simulink model "s5"  (R2023b)
settings: Solver=ode45  StartTime=3  StopTime=10  RelTol=1e-3
settings Model: Creator=t3  LastModifiedBy=t3

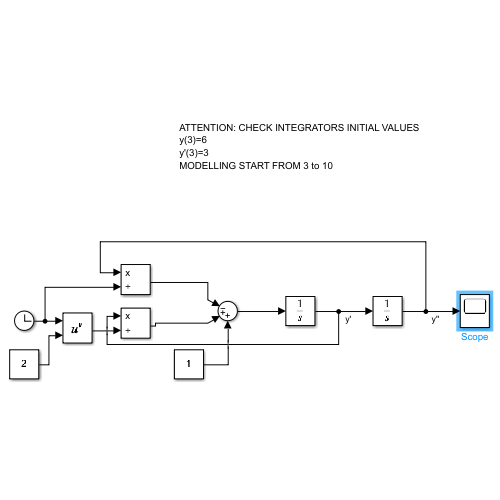
[thumbnail: Simulink's stored preview of the top-level diagram]
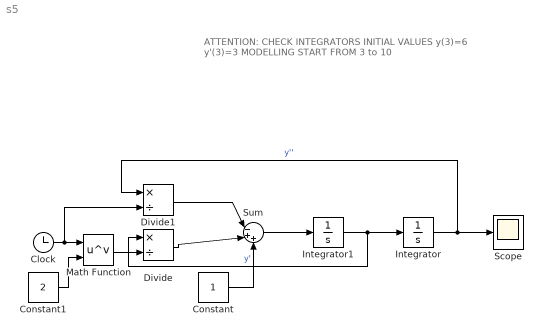
== system s5 ==
  note: ATTENTION: CHECK INTEGRATORS INITIAL VALUES
      | y(3)=6
      | y'(3)=3
      | MODELLING START FROM 3 to 10
  Clock : Clock
  Constant : Constant
  Constant1 : Constant  Value=2
  Divide : Product  Inputs=*/
  Divide1 : Product  Inputs=*/
  Integrator : Integrator  InitialCondition=3
  Integrator1 : Integrator  InitialCondition=6
  Math Function : Math  Operator=pow
  Scope : Scope
  Sum : Sum  Inputs=|-++
  wires:
  Integrator/1 -> Divide1/1, Scope/1  "y''"
  Integrator1/1 -> Divide/1, Integrator/1  "y'"
  Sum/1 -> Integrator1/1
  Constant/1 -> Sum/3
  Divide/1 -> Sum/2
  Divide1/1 -> Sum/1
  Math Function/1 -> Divide/2
  Clock/1 -> Divide1/2, Math Function/1
  Constant1/1 -> Math Function/2
